simulink model "hw3_p1_glider"  (R2020a)
settings: Solver=VariableStepAuto  StartTime=0.0  StopTime=600  RelTol=1e-7
undefined symbols (not defined in the file): CL, h_i, Vh_i, Vx_i, x_i
settings Model: Creator=Tomo  LastModifiedBy=Tomo

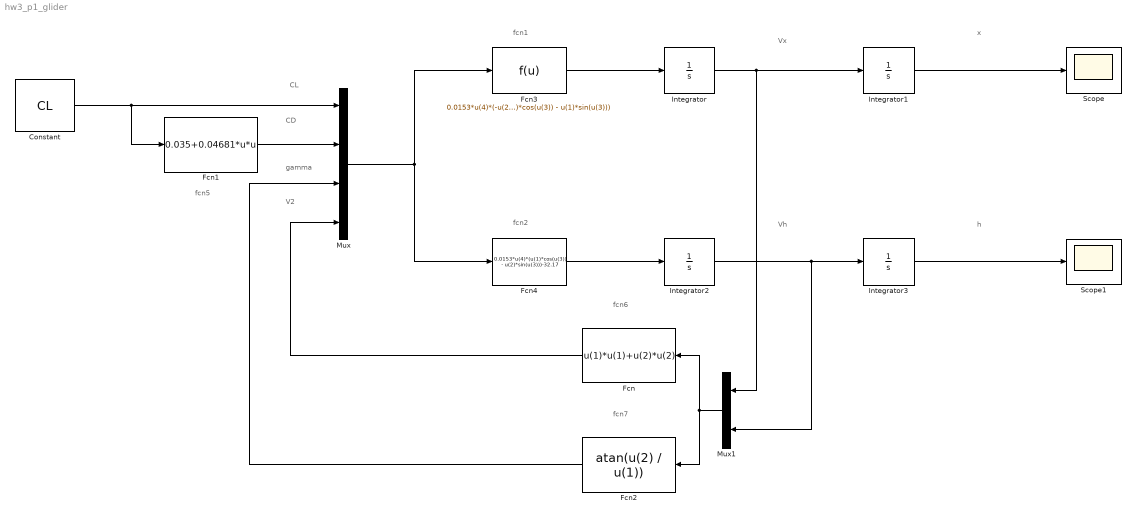
== system hw3_p1_glider ==
  note: fcn1
  note: Vh
  note: CL
  note: x
  note: h
  note: fcn2
  note: fcn6
  note: fcn7
  note: fcn5
  note: CD
  note: gamma
  note: V2
  note: Vx
  Constant : Constant  Value=CL
  Fcn : Fcn  Expr=u(1)*u(1)+u(2)*u(2)
  Fcn1 : Fcn  Expr=0.035+0.04681*u*u
  Fcn2 : Fcn  Expr=atan(u(2) / u(1))
  Fcn3 : Fcn  Expr=0.0153*u(4)*(-u(2)*cos(u(3)) - u(1)*sin(u(3)))
  Fcn4 : Fcn  Expr=0.0153*u(4)*(u(1)*cos(u(3)) - u(2)*sin(u(3)))-32.17
  Integrator : Integrator  InitialCondition=Vx_i
  Integrator1 : Integrator  InitialCondition=x_i
  Integrator2 : Integrator  InitialCondition=Vh_i
  Integrator3 : Integrator  InitialCondition=h_i
  Mux : Mux
  Mux1 : Mux  Inputs=2
  Scope : Scope
  Scope1 : Scope
  wires:
  Constant/1 -> Fcn1/1, Mux/1
  Fcn1/1 -> Mux/2
  Mux/1 -> Fcn4/1, Fcn3/1
  Fcn3/1 -> Integrator/1
  Integrator/1 -> Mux1/1, Integrator1/1
  Fcn4/1 -> Integrator2/1
  Integrator1/1 -> Scope/1
  Integrator3/1 -> Scope1/1
  Mux1/1 -> Fcn/1, Fcn2/1
  Integrator2/1 -> Mux1/2, Integrator3/1
  Fcn/1 -> Mux/4
  Fcn2/1 -> Mux/3
